simulink model "patientModel"  (R2020a)
settings: Solver=VariableStepAuto  StartTime=0.0  StopTime=365  RelTol=1e-3
undefined symbols (not defined in the file or in its folder): normal, prob, sigbuilder_block, startCond
settings Model: Creator=acook  LastModifiedBy=acook

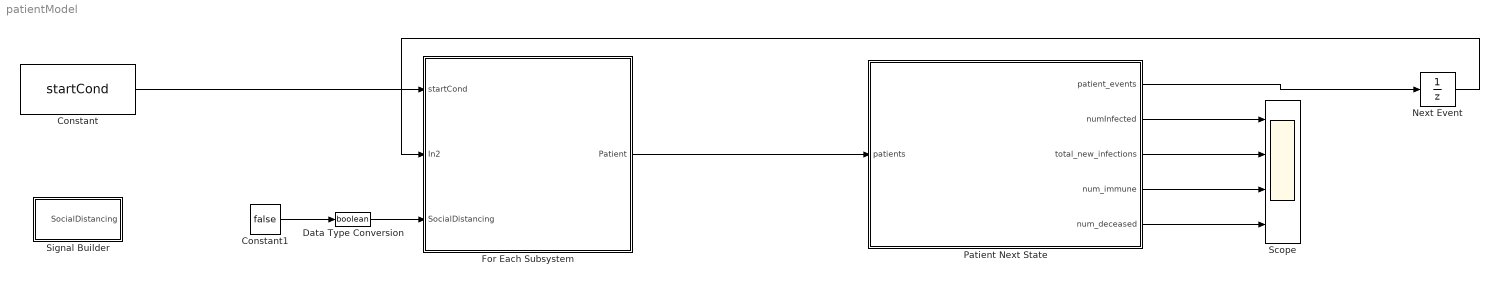
== system patientModel ==
  Constant : Constant  Value=startCond
  Constant1 : Constant  Value=false
  Data Type Conversion : DataTypeConversion  OutDataTypeStr=boolean
  For Each Subsystem : Subsystem  TreatAsAtomicUnit=on
  Next Event : UnitDelay  SampleTime=-1  HasFrameUpgradeWarning=on
  Patient Next State : MATLAB Function  TreatAsAtomicUnit=on
  Scope : Scope  NumInputPorts=4
  Signal Builder : Subsystem  Tag=STV Subsys  LoadFcn=sigbuilder_block('load',[437.6 199.2 550.4 400 ]);  StartFcn=sigbuilder_block('start');  StopFcn=sigbuilder_block('stop');  ClipboardFcn=sigbuilder_block('clipboard');  mask(Sigbuilder block){tuvar=[0:10]}
      mask help: Simulink:masks:SigbuilderBlock_MD
      mask init:
      | if ~strcmp(get_param(bdroot(gcbh),'SimulationStatus'),'stopped') tuvar = sigbuilder_block('maskInit'); end
      settings: CopyFcn=sigbuilder_block('copy');  DeleteFcn=sigbuilder_block('delete');  ModelCloseFcn=sigbuilder_block('modelClose');  PreSaveFcn=sigbuilder_block('preSave');  PauseFcn=sigbuilder_block('pause');  ContinueFcn=sigbuilder_block('continue');  NameChangeFcn=sigbuilder_block('namechange');  OpenFcn=sigbuilder_block('open',[437.6 199.2 550.4 400 ]);  CloseFcn=sigbuilder_block('close');
      mask Display: plot(0, 0, 100, 100,[2, 2, 32, 32, 2], [68, 8, 8, 68, 68],[32, 2], [38, 38], [32, 19, 2],[53, 60, 44], [32, 17, 17, 2],[16, 16, 31, 31]);txt = getActiveGroup(gcbh);text(2, 100, txt,'verticalAlignment', 'top');
  wires:
  For Each Subsystem/1(Patient) -> Patient Next State/1(patients)
  Constant/1 -> For Each Subsystem/1(startCond)
  Patient Next State/1(patient_events) -> Next Event/1
  Next Event/1 -> For Each Subsystem/2(In2)
  Patient Next State/2(numInfected) -> Scope/1
  Patient Next State/3(total_new_infections) -> Scope/2
  Patient Next State/4(num_immune) -> Scope/3
  Patient Next State/5(num_deceased) -> Scope/4
  Constant1/1 -> Data Type Conversion/1
  Data Type Conversion/1 -> For Each Subsystem/3(SocialDistancing)

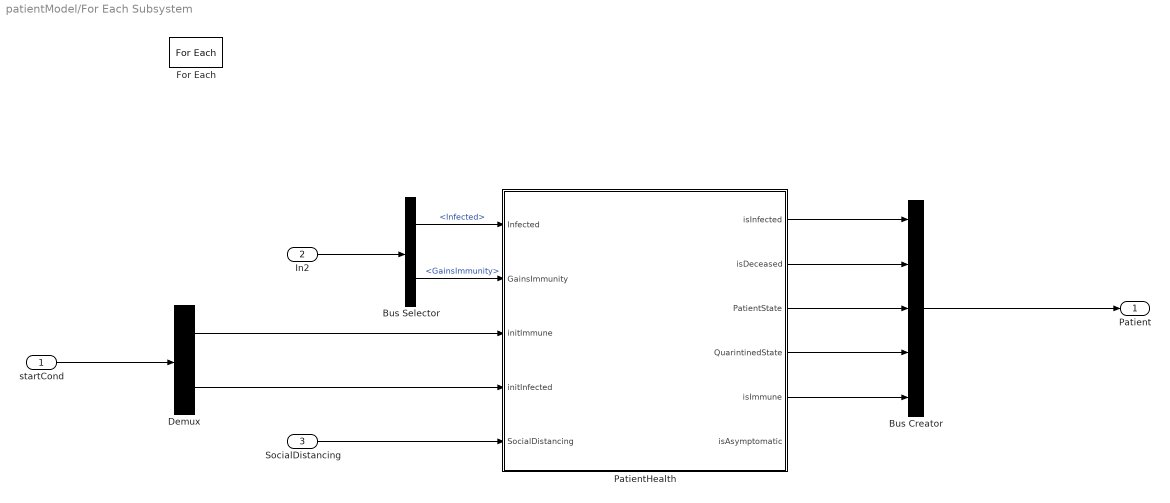
== system patientModel/For Each Subsystem ==
  startCond : Inport  Partition=on  PartitionDimension=2  PartitionWidth=1  PartitionOffset=0
  In2 : Inport  Port=2  Partition=on  PartitionDimension=1  PartitionWidth=1  PartitionOffset=0
  SocialDistancing : Inport  Port=3
  Bus Creator : BusCreator  Inputs=5  OutDataTypeStr=Bus: PatientBus  NonVirtualBus=on
  Bus Selector : BusSelector  OutputSignals=Infected,GainsImmunity
  Demux : Demux  Outputs=2
  For Each : ForEach  DisableCoverage=on
  PatientHealth : Stateflow chart  TreatAsAtomicUnit=on
  Patient : Outport  ConcatenationDimension=1
  wires:
  PatientHealth/5(isImmune) -> Bus Creator/5
  PatientHealth/3(PatientState) -> Bus Creator/3
  PatientHealth/1(isInfected) -> Bus Creator/1
  PatientHealth/4(QuarintinedState) -> Bus Creator/4
  Bus Creator/1 -> Patient/1
  PatientHealth/2(isDeceased) -> Bus Creator/2
  startCond/1 -> Demux/1
  Demux/2 -> PatientHealth/4(initInfected)
  Demux/1 -> PatientHealth/3(initImmune)
  In2/1 -> Bus Selector/1
  Bus Selector/1 -> PatientHealth/1(Infected)  "<Infected>"
  Bus Selector/2 -> PatientHealth/2(GainsImmunity)  "<GainsImmunity>"
  SocialDistancing/1 -> PatientHealth/5(SocialDistancing)

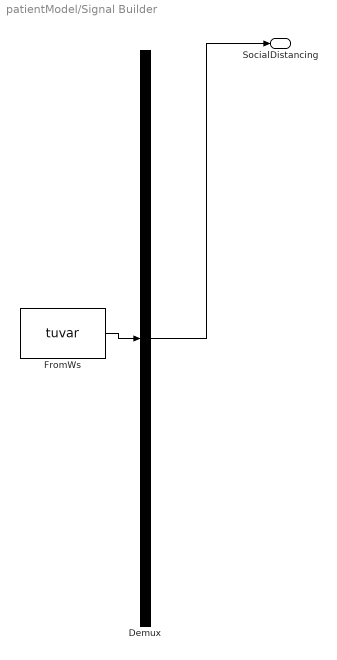
== system patientModel/Signal Builder ==
  Demux : Demux  Tag=STV Demux  Outputs=1
      settings: DisplayOption=none
  FromWs : FromWorkspace  Tag=STV FromWs  VariableName=tuvar
      SigBuilderData=|
      | common.afterFinalStr = 'Extrapolate'
      | common.sampleTime = 0
      | dataSet.timeRange = [0 365]
      | dataSet.name = 'Group 1'
      | sbobj.Groups.Name = 'Group 1'
      | sbobj.Groups.Signals.Name = 'SocialDistancing'
      | sbobj.Groups.Signals.XData = [0 50 50 100 100 365]
      | sbobj.Groups.Signals.YData = [0 0 1 1 0 0]
      | sbobj.Groups.TimeRange = [0 365]
  SocialDistancing : Outport  Tag=STV Outport
  wires:
  FromWs/1 -> Demux/1
  Demux/1 -> SocialDistancing/1

== matlab function patientModel/Patient Next State ==
  data: patients input Bus: PatientBus; patient_events output Bus: PatientEvents; numInfected output; prob parameter; normal parameter; total_new_infections output; num_immune output; num_deceased output
function [patient_events,numInfected,total_new_infections, ...
    num_immune,num_deceased ...
] = fcn(patients, prob, normal)

num_patients = length(patients);
fns = length(fieldnames(patients));

patient_t = table('Size',[length(patients) fns], ...
    'VariableTypes',{'logical' 'logical' 'double' 'double' 'logical'}, ... % This needs to match the bus
    'VariableNames',{'isInfected','isDeceased','PatientState','QuarintineState','isImmune'} ...
    );

% Current State Conversion to table
for row_idx = 1:num_patients
    row_idx;
    patient_t(row_idx,1) = {patients(row_idx).isInfected};
    patient_t(row_idx,2) = {patients(row_idx).isDeceased};
    patient_t(row_idx,3) = {double(patients(row_idx).PatientState)};
    patient_t(row_idx,4) = {double(patients(row_idx).QuarintineState)};
    patient_t(row_idx,5) = {patients(row_idx).isImmune};
end

% Next state initalization
pinit.Infected = false;
pinit.GainsImmunity = false;
patient_events = repmat(pinit,num_patients,1);


% Get the infected patients
p_infected = patient_t(patient_t.isInfected,:);
isHealthy = ~patient_t.isInfected;

numInfected = height(p_infected);

boolInfected = false(num_patients,1);

% Roll to infect new patients
for row_idx = 1:height(p_infected)
    
    % Get the quarintine level
    qlvl = EnumQuarintine(p_infected.QuarintineState(row_idx));
    switch qlvl
        case EnumQuarintine.None;                       interaction_prob = normal.interaction.None;
        case EnumQuarintine.Full;                          interaction_prob = normal.interaction.Full;
        case EnumQuarintine.Medical;                    interaction_prob = normal.interaction.Medical;
        case EnumQuarintine.SociallyDistanced;    interaction_prob = normal.interaction.SociallyDistanced;
        otherwise
            error('Bad value for EnumQuarintine');
    end
    
    interactions = round(norm_dist(interaction_prob));
    
    new_infections = roll_dice_tf(prob.infection_chance,interactions);
    
    if new_infections > 0
        % Randomly infect uninfected
        idx_healthy = find(isHealthy == 1); % Find indexes of health people only
        if length(idx_healthy) > 1 % if there are healthy people to infect
            idx_infect = randsample(idx_healthy,new_infections); % Randomly infect the healthy
            boolInfected(idx_infect) = true;
        end
    end
    
end

total_new_infections = sum(boolInfected);

for idx = 1:num_patients
    patient_events(idx).Infected = boolInfected(idx);
end

%% Statiscal outputs
num_immune   = height(patient_t(patient_t.isImmune,:));
num_deceased = height(patient_t(patient_t.isImmune,:));

end


function dist = norm_dist(ary)
%% Array [mu sigma]
dist = normrnd(ary(1),ary(2));
end


function [total, sel] = roll_dice_tf(chance,Nroll)
% Chance - probability of getting true
% Nroll - Number of times to roll
val = [true false];
r = rand(Nroll,1) < chance;
sel = val(2 - r); % use as index into VAL
total = sum(sel);
end

== stateflow chart patientModel/For Each Subsystem/PatientHealth ==
  state Health [parallel]
    settings: executionOrder=2
    state Initial
      PatientState = Healthy;
      QuarintinedState = None;
      isDeceased = false;
      isImmune = initImmune;
      isInfected = initInfected;
      isAsymptomatic = false;
      isDiagnosed = false;
    state Immune
      PatientState = Immune;
      isImmune = true;
    state Healthy
      PatientState = Healthy;
    state Carrier
      en:
      PatientState = Carrier;
      isInfected = true;
      isDiagnosed = false;
      isAsymptomatic = flat_dist(prob.asymptomatic)
      tSymptoms = norm_dist(normal.symptom_time);
      isFatal = flat_dist(prob.fatality);
      tInfected = norm_dist(normal.infection_time);
      ex:
      isInfected = false;
      isDiagnosed = false;
      du:
      state NoSymptoms
      state Symptoms
        en: isDiagnosed = flat_dist(prob.diagnose)
      (default) -> NoSymptoms
      NoSymptoms -> Symptoms : [~isAsymptomatic && after(tSymptoms,tick)]
    state Deceased
      PatientState = Deceased;
      isDeceased = true;
    (default) -> Initial
    Initial -> (junction 41)
    (junction 41) -> (junction 44) [order 1] : [isImmune]
    (junction 41) -> Healthy [order 2]
    (junction 44) -> Immune
    (junction 50) -> Immune
    (junction 48) -> Healthy [order 2]
    (junction 48) -> (junction 50) [order 1] : [GainsImmunity]
    (junction 34) -> (junction 48) [order 2]
    Healthy -> Carrier : [Infected]
    Carrier -> (junction 34) : after(tInfected,tick)
    (junction 34) -> Health.Deceased [order 1] : [isFatal]
  state QuarintineLevel [parallel]
    settings: executionOrder=1
    state Alive
      state Start
        QuarintinedState = None;
      state Medical
        QuarintinedState = Medical;
      state SocialDistancing
        QuarintinedState = SociallyDistanced;
      Start -> (junction 88) [order 1] : [isInfected && isDiagnosed]
      (junction 88) -> Medical
      Start -> SocialDistancing [order 2] : [SocialDistancing]
      Medical -> Start : [~isInfected]
      (junction 90) -> Medical
      SocialDistancing -> (junction 90) : [isInfected && isDiagnosed]
    state Deceased
      QuarintinedState = Full;
    (default) -> Start
    Alive -> QuarintineLevel.Deceased : [isDeceased]
  data: ary function_input; dist function_output; per function_input; dist function_output; isInfected output; Infected input; GainsImmunity input; isDeceased output; PatientState output Enum: EnumPatient; QuarintinedState output Enum: EnumQuarintine; isImmune output; initImmune input; initInfected input; SocialDistancing input; isAsymptomatic output; prob parameter; isDiagnosed local; tSymptoms local; normal parameter; isFatal local; tInfected local
  function dist = norm_dist(ary):
    | function dist = norm_dist(ary)
    | %% Array [mu sigma]
    | dist = normrnd(ary(1),ary(2),1);
    | end
  function dist = flat_dist(per):
    | function dist = flat_dist(per)
    | dist = rand < per;
    | end
